simulink model "pd"  (R2018a)
settings: Solver=VariableStepAuto  StartTime=0.0  StopTime=10.0  RelTol=1e-3
undefined symbols (not defined in the file): KKt, Kt
settings Model: Creator=eechris  LastModifiedBy=eechris

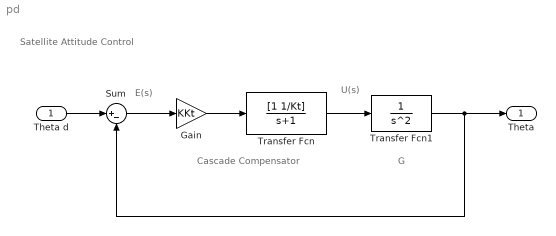
== system pd ==
  note: U(s)
  note: E(s)
  note: G
  note: Cascade Compensator
  note: Satellite Attitude Control
  Theta d : Inport
  Gain : Gain  Gain=KKt
  Sum : Sum  Inputs=|+-
  Transfer Fcn : TransferFcn  Numerator=[1 1/Kt]  Denominator=[1 1]
  Transfer Fcn1 : TransferFcn  Denominator=[1 0 0]
  Theta : Outport
  wires:
  Transfer Fcn/1 -> Transfer Fcn1/1
  Theta d/1 -> Sum/1
  Transfer Fcn1/1 -> Sum/2, Theta/1
  Gain/1 -> Transfer Fcn/1
  Sum/1 -> Gain/1
